simulink model "pid_1"  (R2025b)
settings: Solver=VariableStepAuto  StartTime=0.0  StopTime=inf  RelTol=1e-3
libraries: opcualib x2, slpidlib x1, simulink x1
settings Model: Creator=Maksim  LastModifiedBy=Maksim

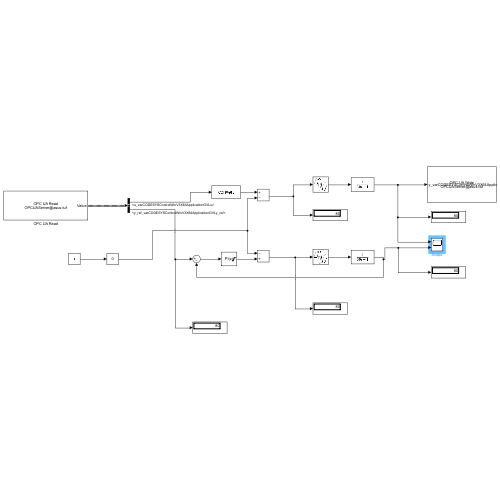
[thumbnail: Simulink's stored preview of the top-level diagram]
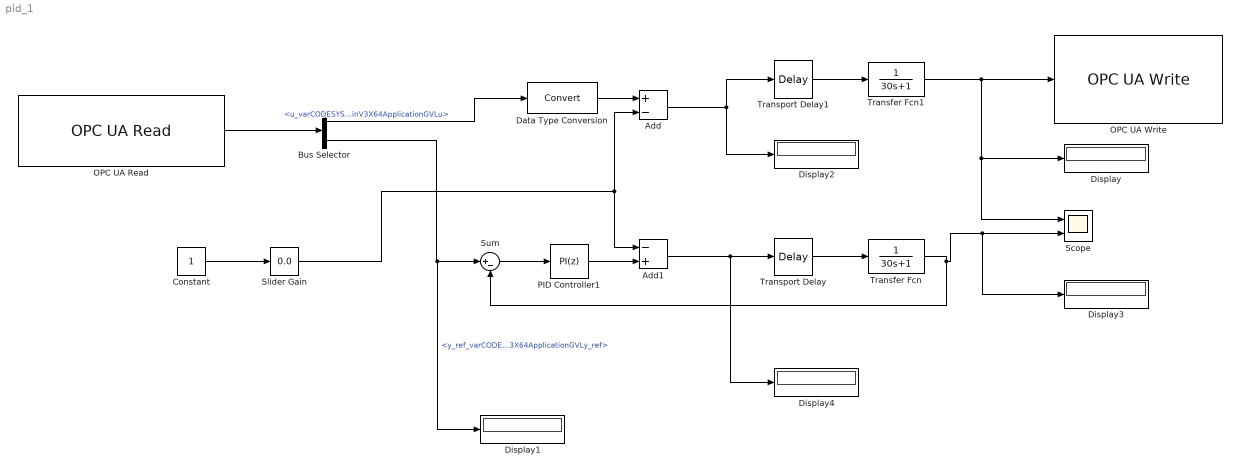
== system pid_1 ==
  Add : Sum  Inputs=+-
  Add1 : Sum  Inputs=-+
  Bus Selector : BusSelector  OutputSignals=u_varCODESYSControlWinV3X64ApplicationGVLu,y_ref_varCODESYSControlWinV3X64ApplicationGVLy_ref
  Constant : Constant
  Data Type Conversion : DataTypeConversion  SaturateOnIntegerOverflow=off  RndMeth=Floor
  Display{,1..4} (5 alike) : Display
      Display1 settings: Tag=Setpoint  Description=Setpoint
      Display2 settings: Tag=Setpoint  Description=Setpoint
      Display3 settings: Tag=Setpoint  Description=Setpoint
      Display4 settings: Tag=Setpoint  Description=Setpoint
  OPC UA Read : opcualib/OPC UA Read  SelectedServer=OPCUAServer@asus-tuf  ServerList=OPCUAServer@asus-tuf  NodeList={ '1', 'u', '4', '|var|CODESYS Control Win V3 x64.Application.GVL.u', '0'; '2', 'y_ref', '4', '|var|CODESYS Control Win V3 x64.Application.GVL.y_ref', '0' }  ShowQualityPort=off  ShowTimestampPort=off  ShowTimestampPortAs=Seconds since start  SampleTime=-1
  OPC UA Write : opcualib/OPC UA Write  SelectedServer=OPCUAServer@asus-tuf  ServerList=OPCUAServer@asus-tuf  SampleTime=-1  NodeList={ '1', 'y', '4', '|var|CODESYS Control Win V3 x64.Application.GVL.y', '0' }
  PID Controller1 : slpidlib/PID Controller  Controller=PI  Form=Ideal  TimeDomain=Discrete-time  UseExternalTs=off  SampleTime=1  IntegratorMethod=Forward Euler  FilterMethod=Forward Euler  ControllerParametersSource=internal  P=1.65  I=0.05  UseKiTs=off  D=0.32  UseExternalDerivativeSource=off  N=100  UseFilter=on  TunerSelectOption=Transfer Function Based (PID Tuner App)  InitialConditionSource=internal  InitialConditionForIntegrator=0  InitialConditionForFilter=0  DifferentiatorICPrevScaledInput=0  ExternalReset=none  TrackingMode=off  Kt=1  LimitOutput=on  SatLimitsSource=internal  UpperSaturationLimit=100  LowerSaturationLimit=0  LinearizeAsGain=on  AntiWindupMode=clamping  Kb=1  LimitIntegrator=off  UpperIntegratorSaturationLimit=inf  LowerIntegratorSaturationLimit=-inf  POutMin=[]  POutMax=[]  IOutMin=[]  IOutMax=[]  DOutMin=[]  DOutMax=[]  NOutMin=[]  NOutMax=[]  SumOutMin=[]  SumOutMax=[]  SaturationOutMin=[]  SaturationOutMax=[]  PParamMin=[]  PParamMax=[]  IParamMin=[]  IParamMax=[]  DParamMin=[]  DParamMax=[]  NParamMin=[]  NParamMax=[]  KbParamMin=[]  KbParamMax=[]  KtParamMin=[]  KtParamMax=[]  KbOutMin=[]  KbOutMax=[]  KtOutMin=[]  KtOutMax=[]  IntegratorOutMin=[]  IntegratorOutMax=[]  FilterOutMin=[]  FilterOutMax=[]  SumI1OutMin=[]  SumI1OutMax=[]  SumI2OutMin=[]  SumI2OutMax=[]  SumI3OutMin=[]  SumI3OutMax=[]  SumI4OutMin=[]  SumI4OutMax=[]  SumDOutMin=[]  SumDOutMax=[]  DifferentiatorOutMin=[]  DifferentiatorOutMax=[]  FilterDiffOutCoefMin=[]  FilterDiffOutCoefMax=[]  ReciprocalOutMin=[]  ReciprocalOutMax=[]  SumDenOutMin=[]  SumDenOutMax=[]  SumNumOutMin=[]  SumNumOutMax=[]  DivideOutMin=[]  DivideOutMax=[]  UdiffTsProdOutMin=[]  UdiffTsProdOutMax=[]  NTsProdOutMin=[]  NTsProdOutMax=[]  UintegralTsProdOutMin=[]  UintegralTsProdOutMax=[]  UngainTsProdOutMin=[]  UngainTsProdOutMax=[]  ClampingZeroOutDataTypeStr=Inherit: Inherit via back propagation  ClampingZeroOutMin=[]  ClampingZeroOutMax=[]  FilterDenConstantOutDataTypeStr=Inherit: Inherit via back propagation  FilterDenConstantOutMin=[]  FilterDenConstantOutMax=[]  PCopyOutDataTypeStr=Inherit: Inherit via back propagation  PCopyOutMin=[]  PCopyOutMax=[]  NCopyOutDataTypeStr=Inherit: Inherit via back propagation  NCopyOutMin=[]  NCopyOutMax=[]  IntegratorContinuousStateAttributes=''  IntegratorStateMustResolveToSignalObject=off  IntegratorRTWStateStorageClass=Auto  FilterContinuousStateAttributes=''  FilterStateMustResolveToSignalObject=off  FilterRTWStateStorageClass=Auto  ParallelPVariant=Passthrough  IdealPVariant=InternalParameters  IVariant=InternalParameters  DVariant=Disabled  IntegratorVariant=Discrete  SatVariant=Enabled  AWVariant=DiscClampingIdeal  PCopyVariant=InternalParamsIdeal  TRVariant=Disabled  FdbkBlocksVariant=Forward  IdealPFdbkVariant=Disabled  SatFdbkVariant=Disabled  DerivativeFilterVariant=Disabled  NVariant=Disabled  NCopyVariant=Disabled_SignalSpec  FilterICVariant=Disabled  IntegratorICVariant=InternalICs  ExternalResetVariant=Disabled  TRSumVariant=Passthrough  SumFdbkVariant=Disabled  SumVariant=Sum_PI  TsampFilterVariant=InternalTs  TsampNgainVariant=Passthrough  TsampIntegralVariant=Disabled_SignalSpec  ExternalSaturationOutDataTypeStr=Inherit: Same as second input  DerivativeSourceVariant=Disabled  PreIntVariant=InternalPreInt
  Scope : Scope  NumInputPorts=2
      settings: ActiveDisplayYMinimum=-354.31116002447112  ActiveDisplayYMaximum=493.89823853236038
  Slider Gain : simulink/Math Operations/Slider Gain  gain=0.0  low=0  high=30
  Sum : Sum  Inputs=|+-
  Transfer Fcn : TransferFcn  Denominator=[30 1]
  Transfer Fcn1 : TransferFcn  Denominator=[30 1]
  Transport Delay : TransportDelay  DelayTime=10  BufferSize=4000
  Transport Delay1 : TransportDelay  DelayTime=10  BufferSize=4000
  wires:
  Transfer Fcn/1 -> Display3/1, Scope/2, Sum/2
  Transport Delay/1 -> Transfer Fcn/1
  Transfer Fcn1/1 -> Scope/1, Display/1, OPC UA Write/1
  Transport Delay1/1 -> Transfer Fcn1/1
  Sum/1 -> PID Controller1/1
  OPC UA Read/1 -> Bus Selector/1
  Bus Selector/2 -> Display1/1, Sum/1  "<y_ref_varCODESYSControlWinV3X64ApplicationGVLy_ref>"
  Bus Selector/1 -> Data Type Conversion/1  "<u_varCODESYSControlWinV3X64ApplicationGVLu>"
  Data Type Conversion/1 -> Add/1
  Add/1 -> Transport Delay1/1, Display2/1
  PID Controller1/1 -> Add1/2
  Add1/1 -> Display4/1, Transport Delay/1
  Slider Gain/1 -> Add1/1, Add/2
  Constant/1 -> Slider Gain/1
